simulink model "apilot1"  (Simulink 2.09)
settings: Solver=ode15s  StartTime=0.0  StopTime=100  MaxStep=2  RelTol=1e-06  AbsTol=1e-04
values from neighbouring files (symbols this model uses):
  ymod1A = [1 1 1 0 0]'    [apmode.m]
  ymod1S = [1 1 1 0 0]'    [apmode.m]
  yrefA = [0 Dpsir]'    [apmode.m]
  yrefS = [0 0 DHdotr]'    [apmode.m]
undefined symbols (not defined in the file or in its folder): Aail, Aelv, AM, Arud, Bail, Belv, Brud, Cail, Celv, Crud, Dail, Delv, Drud, GM1, sfunyst, uaero0, uprop0, xdot0, xfix, xinco
(part 1 of 2)
settings Model: SaveTime=off  SaveOutput=off  ConsistencyChecking=off  RTWTemplateMakefile=grt_vc.tmf

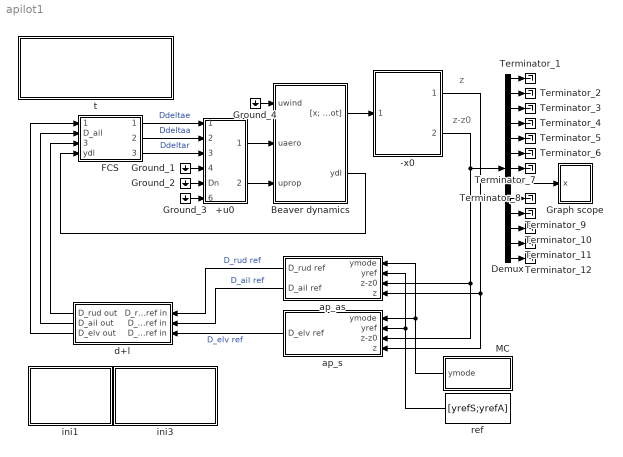
== system apilot1 ==
  note: z-z0
  note: z
  +u0 : Subsystem
      mask Display: disp('Add\ninitial\ninputs')
  -x0 : Subsystem
      mask Display: disp('Subtract\ninitial con-\nditions\n\nNo sensors!')
  Beaver dynamics : Subsystem
  Demux : Demux  Outputs=13
  FCS : Subsystem
      mask Display: disp('Actuator &\ncable dy-\nnamics')
  Graph scope : Subsystem  mask(Storage scope.){npts=100, color='g-'}
      mask prompts: npts "Initial Time Range:"; color "Initial y-min:"
      mask help:
      | Storage scope using MATLAB graph window.
      | Enter plotting ranges and line type.
      mask init:
      | close all; ax = [0, @1, @2, @3];
      mask Help: Uses MATLAB's graph window.\nUse only one block per system.\nLine type must be in quotes.\nSee the M-file sfunyst.m.
      mask Display: plot(0,0,100,100,[83,76,63,52,42,38,28,16,11,84,11,11,11,90,90,11],[75,58,47,54,72,80,84,74,65,65,65,90,40,40,90,90])
  Ground_{1..4} (4 alike) : Ground
  MC : Subsystem  Orientation=left
      mask Display: disp('Mode\nController')
  Terminator_{1..12} (12 alike) : Terminator
  ap_as : Subsystem  Orientation=left
      mask Display: disp('Asymmetrical\nautopilot modes')
  ap_s : Subsystem  Orientation=left
      mask Display: disp('Symmetrical\nautopilot modes')
  d+l : Subsystem  Orientation=left
      mask Display: disp('computational\ndelay & limiters')
  ini1 : Subsystem
      settings: OpenFcn=apinit
      mask Type: apinit
      mask Display: disp('1. Initialize\nsubsystems\n\nAPINIT')
  ini3 : Subsystem
      settings: OpenFcn=apmode
      mask Type: apmode
      mask Display: disp('2. Select mode &\nreference signals\n\nAPMODE')
  ref : Constant  Orientation=left  Value=[yrefS;yrefA]
      mask Display: disp('Reference\nsignals')
  t : Subsystem
      settings: OpenFcn=fdchelp apilot
      mask Display: disp('Apilot1 (no radio-navigation,\nwind, turbulence, and\nsensor models)\nMarc Rauw, June 2000')
  wires:
  +u0/2(uprop) -> Beaver dynamics/3(uprop)
  +u0/1(uaero) -> Beaver dynamics/2(uaero)
  Beaver dynamics/1("[x; Hdot]") -> -x0/1("[x; Hdot]")
  FCS/3(Ddeltar) -> +u0/3(Ddeltar)  "Ddeltar"
  FCS/2(Ddeltaa) -> +u0/2(Ddeltaa)  "Ddeltaa"
  FCS/1(Ddeltae) -> +u0/1(Ddeltae)  "Ddeltae"
  d+l/1(D_rud out) -> FCS/3(D_rud)
  d+l/2(D_ail out) -> FCS/2(D_ail)
  d+l/3(D_elv out) -> FCS/1(D_elv)
  ap_s/1(D_elv ref) -> d+l/3(D_elv ref in)  "D_elv ref"
  -x0/1("z == [x; Hdot] ") -> ap_s/4(z), ap_as/4(z)
  ref/1 -> ap_as/2(yref), ap_s/2(yref)
  -x0/2(z-z0 == [x-x0; Hdot-Hdot0]) -> ap_s/3(z-z0), ap_as/3(z-z0), Demux/1
  ap_as/1(D_rud ref) -> d+l/1(D_rud ref in)  "D_rud ref"
  ap_as/2(D_ail ref) -> d+l/2(D_ail ref in)  "D_ail ref"
  Beaver dynamics/2(ydl) -> FCS/4(ydl)
  MC/1(ymode) -> ap_as/1(ymode), ap_s/1(ymode)
  Demux/8 -> Graph scope/1(x)
  Ground_1/1 -> +u0/4(Ddeltaf)
  Ground_2/1 -> +u0/5(Dn)
  Ground_3/1 -> +u0/6(Dpz)
  Demux/1 -> Terminator_1/1
  Demux/2 -> Terminator_2/1
  Demux/3 -> Terminator_3/1
  Demux/4 -> Terminator_4/1
  Demux/5 -> Terminator_5/1
  Demux/6 -> Terminator_6/1
  Demux/7 -> Terminator_7/1
  Demux/9 -> Terminator_8/1
  Demux/10 -> Terminator_9/1
  Demux/11 -> Terminator_10/1
  Demux/12 -> Terminator_11/1
  Demux/13 -> Terminator_12/1
  Ground_4/1 -> Beaver dynamics/1(uwind)

== system apilot1/+u0 ==
  note: Add initial inputs
  note: ENGINE INPUTS:
  note: AERODYNAMIC INPUTS:
  Ddeltae : Inport  Port=1  PortWidth=-1  SampleTime=-1
  Ddeltaa : Inport  Port=2  PortWidth=-1  SampleTime=-1
  Ddeltar : Inport  Port=3  PortWidth=-1  SampleTime=-1
  Ddeltaf : Inport  Port=4  PortWidth=-1  SampleTime=-1
  Dn : Inport  Port=5  PortWidth=-1  SampleTime=-1
  Dpz : Inport  Port=6  PortWidth=-1  SampleTime=-1
  Initial inputs for aeromod : Constant  Value=uaero0
  Initial inputs for engmod : Constant  Value=uprop0
  Mux1 : Mux  Inputs=4
  Mux2 : Mux  Inputs=2
  Sum : Sum  Inputs=++
  Sum1 : Sum  Inputs=++
  uaero : Outport  Port=1  InitialOutput=0
  uprop : Outport  Port=2  InitialOutput=0
  wires:
  Dpz/1 -> Mux2/2
  Dn/1 -> Mux2/1
  Initial inputs for engmod/1 -> Sum/2
  Mux2/1 -> Sum/1
  Sum/1 -> uprop/1
  Ddeltaa/1 -> Mux1/2
  Ddeltae/1 -> Mux1/1
  Ddeltar/1 -> Mux1/3
  Ddeltaf/1 -> Mux1/4
  Initial inputs for aeromod/1 -> Sum1/1
  Sum1/1 -> uaero/1
  Mux1/1 -> Sum1/2

== system apilot1/-x0 ==
  note: Subtract initial conditions
  "[x; Hdot]" : Inport  Port=1  PortWidth=-1  SampleTime=-1
  Initial condition : Constant  Value=[xinco; xdot0(12)]
  Sum : Sum  Inputs=+-
  "z == [x; Hdot] " : Outport  Port=1  InitialOutput=0
  z-z0 == [x-x0; Hdot-Hdot0] : Outport  Port=2  InitialOutput=0
  wires:
  "[x; Hdot]"/1 -> "z == [x; Hdot] "/1, Sum/1
  Initial condition/1 -> Sum/2
  Sum/1 -> z-z0 == [x-x0; Hdot-Hdot0]/1

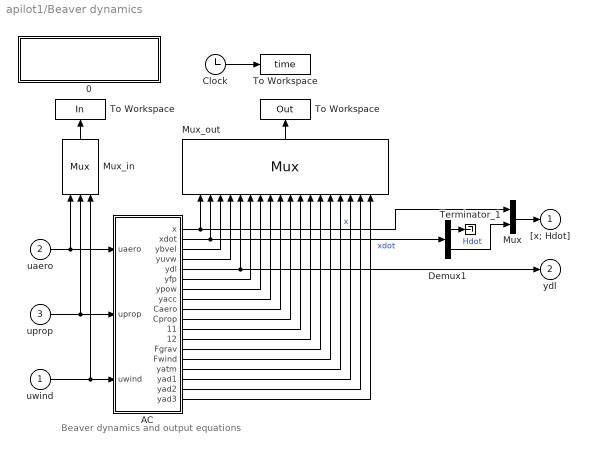
== system apilot1/Beaver dynamics ==
  note: Beaver dynamics
      | and output equations
  uwind : Inport  Port=1  PortWidth=6  SampleTime=-1
  uaero : Inport  Port=2  PortWidth=4  SampleTime=-1
  uprop : Inport  Port=3  PortWidth=2  SampleTime=-1
  0 : Subsystem
      settings: OpenFcn=fdchelp level1
      mask Display: disp('Subsystem equivalent of\nthe S-function BEAVER\nM.O. Rauw, October 1997')
  AC : Subsystem
  Clock : Clock
  Demux1 : Demux  Outputs=[11 1]
  Mux : Mux  Inputs=[12 1]
  Mux_in : Mux  Orientation=up  Inputs=[4 2 6]
      settings: OpenFcn=fdchelp inputs
      mask Display: disp('Mux\nclick\n2x for\ninfo!')
  Mux_out : Mux  Orientation=up  Inputs=[12 12 3 3 3 4 2 6 6 6 6 6 3 3 5 3 3 3]
      settings: OpenFcn=fdchelp outputs
      mask Display: disp('Mux\n\nDouble-click for info!')
  Terminator_1 : Terminator
  To Workspace : ToWorkspace  VariableName=Out  SampleTime=0
      settings: Orientation=up  Buffer=5000
  "To Workspace " : ToWorkspace  VariableName=In  SampleTime=0
      settings: Orientation=up  Buffer=5000
  "To Workspace  " : ToWorkspace  VariableName=time  SampleTime=0
      settings: Buffer=5000
  "[x; Hdot]" : Outport  Port=1  InitialOutput=0
  ydl : Outport  Port=2  InitialOutput=0
  wires:
  AC/7(ypow) -> Mux_out/7
  Mux_in/1 -> "To Workspace "/1
  Mux_out/1 -> To Workspace/1
  Clock/1 -> "To Workspace  "/1
  AC/2(xdot) -> Mux_out/2, Demux1/1  "xdot"
  AC/15(yatm) -> Mux_out/15
  AC/14(Fwind) -> Mux_out/14
  AC/13(Fgrav) -> Mux_out/13
  AC/12(FMprop) -> Mux_out/12
  AC/11(FMaero) -> Mux_out/11
  AC/10(Cprop) -> Mux_out/10
  AC/9(Caero) -> Mux_out/9
  AC/8(yacc) -> Mux_out/8
  AC/6(yfp) -> Mux_out/6
  AC/5(ydl) -> ydl/1, Mux_out/5
  AC/16(yad1) -> Mux_out/16
  AC/3(ybvel) -> Mux_out/3
  AC/1(x) -> Mux/1, Mux_out/1  "x"
  AC/4(yuvw) -> Mux_out/4
  AC/17(yad2) -> Mux_out/17
  AC/18(yad3) -> Mux_out/18
  uwind/1 -> AC/3(" uwind"), Mux_in/3
  uprop/1 -> AC/2(uprop), Mux_in/2
  uaero/1 -> AC/1(uaero), Mux_in/1
  Demux1/1 -> Terminator_1/1
  Demux1/2 -> Mux/2  "Hdot"
  Mux/1 -> "[x; Hdot]"/1

== system apilot1/FCS ==
  note: Actuators
      | + cables:
  D_elv : Inport  Port=1  PortWidth=-1  SampleTime=-1
  D_ail : Inport  Port=2  PortWidth=-1  SampleTime=-1
  D_rud : Inport  Port=3  PortWidth=-1  SampleTime=-1
  ydl : Inport  Port=4  PortWidth=-1  SampleTime=-1
  Demux1 : Demux  Outputs=3
  Mux1 : Mux  Inputs=2
  Mux2 : Mux  Inputs=2
  Mux3 : Mux  Inputs=2
  ailerons : StateSpace  A=Aail  B=Bail  C=Cail*2  D=Dail  X0=0
  elevator : StateSpace  A=Aelv  B=Belv  C=Celv  D=Delv  X0=0
  rudder : StateSpace  A=Arud  B=Brud  C=Crud  D=Drud  X0=0
  t : Subsystem
      settings: OpenFcn=fdchelp actuatr
      mask Display: disp('Actuator & cable dynamics\nMarc Rauw, October 1997')
  Ddeltae : Outport  Port=1  InitialOutput=0
  Ddeltaa : Outport  Port=2  InitialOutput=0
  Ddeltar : Outport  Port=3  InitialOutput=0
  wires:
  Demux1/2 -> Mux1/2
  Demux1/1 -> Mux2/2
  Demux1/3 -> Mux3/2
  Mux1/1 -> elevator/1
  Mux2/1 -> ailerons/1
  Mux3/1 -> rudder/1
  elevator/1 -> Ddeltae/1
  ailerons/1 -> Ddeltaa/1
  ydl/1 -> Demux1/1
  rudder/1 -> Ddeltar/1
  D_elv/1 -> Mux1/1
  D_ail/1 -> Mux2/1
  D_rud/1 -> Mux3/1

== system apilot1/Graph scope ==
  x : Inport  Port=1  PortWidth=-1  SampleTime=-1
  "S-function M-file which plots lines " : S-Function  LoadFcn=sfunyst([],[],[],'LoadBlock')  FunctionName=sfunyst  Parameters=ax, color, npts
      settings: CopyFcn=sfunyst([],[],[],'CopyBlock')  DeleteFcn=sfunyst([],[],[],'DeleteBlock')
  wires:
  x/1 -> "S-function M-file which plots lines "/1

== system apilot1/MC ==
  Mux1 : Mux  Inputs=[5 5]
  asymm. mode-switches : Constant  Value=ymod1A
  symm. mode-switches : Constant  Value=ymod1S
  t : Subsystem
      settings: OpenFcn=fdchelp modectrl
      mask Display: disp('Mode Controller (Mode Select)\nNo on-line mode-switching!\nMarc Rauw, June 2000')
  ymode : Outport  Port=1  InitialOutput=0
  wires:
  symm. mode-switches/1 -> Mux1/1
  Mux1/1 -> ymode/1
  asymm. mode-switches/1 -> Mux1/2

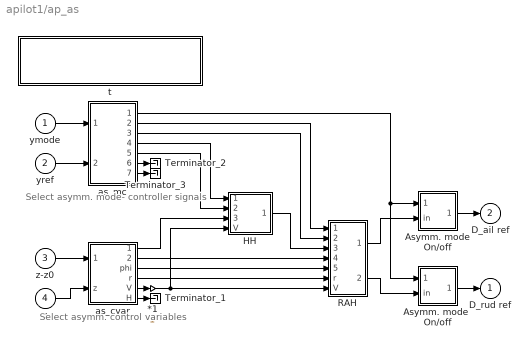
== system apilot1/ap_as ==
  note: Select asymm. mode-
      | controller signals
  note: Select asymm.
      | control variables
  ymode : Inport  Port=1  PortWidth=-1  SampleTime=-1
  yref : Inport  Port=2  PortWidth=-1  SampleTime=-1
  z-z0 : Inport  Port=3  PortWidth=-1  SampleTime=-1
  z : Inport  Port=4  PortWidth=-1  SampleTime=-1
  *1 : Gain  Gain=1
  Asymm. mode On/off : Subsystem
      mask Type: On/off switch
      mask Description:
      | If input(1) = 1
      |      output = input(2)
      |  else if input(1) = 0
      |      output = 0
      mask Help: On/off switch.
      mask Display: plot(0,0,100,100,[31,31,32,34,34,32,31,31,0],[50,48,47,48,51,53,51,50,50],[100,75,51],[50,50,97]);disp('?')
  Asymm. mode  On/off : Subsystem
      mask Type: On/off switch
      mask Description:
      | If input(1) = 1
      |      output = input(2)
      |  else if input(1) = 0
      |      output = 0
      mask Help: On/off switch.
      mask Display: plot(0,0,100,100,[31,31,32,34,34,32,31,31,0],[50,48,47,48,51,53,51,50,50],[100,75,51],[50,50,97]);disp('?')
  HH : Subsystem
  RAH : Subsystem
  Terminator_1 : Terminator
  Terminator_2 : Terminator
  Terminator_3 : Terminator
  as_cvar : Subsystem
  as_mc : Subsystem
  t : Subsystem
      settings: OpenFcn=fdchelp ap_asymm
      mask Display: disp('Asymm. autopilot modes\n(without NAV and LOC modes)\nMarc Rauw, October 1997')
  D_rud ref : Outport  Port=1  InitialOutput=0
  D_ail ref : Outport  Port=2  InitialOutput=0
  wires:
  *1/1 -> RAH/7(V), HH/4(V)
  RAH/2(D_rud ref) -> Asymm. mode  On/off/2(in)
  ymode/1 -> as_mc/1(ymode)
  yref/1 -> as_mc/2(yref)
  Asymm. mode On/off/1(out) -> D_ail ref/1
  Asymm. mode  On/off/1(out) -> D_rud ref/1
  z-z0/1 -> as_cvar/1(z-z0)
  as_cvar/5(V) -> *1/1
  as_cvar/2(phi-phi0) -> RAH/4(phi-phi0)
  as_cvar/3(phi) -> RAH/5(phi)
  as_cvar/4(r) -> RAH/6(r)
  z/1 -> as_cvar/2(z)
  HH/1(Dphir (HH)) -> RAH/3(Dphir (out. loop))
  as_cvar/1(psi-psi0) -> HH/3(psi-psi0)
  RAH/1(D_ail ref) -> Asymm. mode On/off/2(in)
  as_mc/1(asymm. mode?) -> Asymm. mode  On/off/1(crit), Asymm. mode On/off/1(crit)
  as_mc/2(asymm. out. loop?) -> RAH/1(Asymm out. loop?)
  as_mc/3(Dphir (RAH)) -> RAH/2(Dphir (RAH))
  as_mc/4(HH?) -> HH/1(HH?)
  as_mc/5(Dpsir (HH)) -> HH/2(Dpsir (HH))
  as_cvar/6(H) -> Terminator_1/1
  as_mc/6(NAV?) -> Terminator_2/1
  as_mc/7(LOC coupled?) -> Terminator_3/1

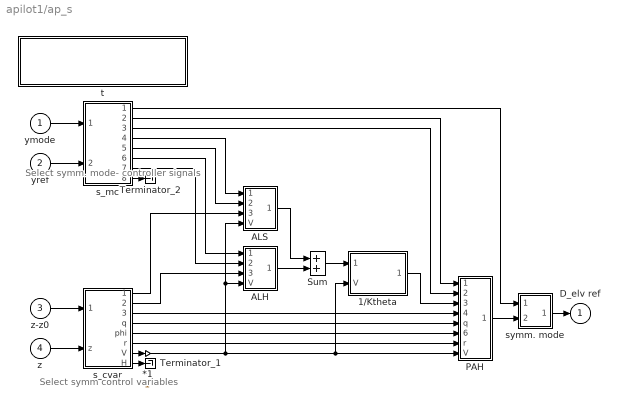
== system apilot1/ap_s ==
  note: Select symm
      | control variables
  note: Select symm. mode-
      | controller signals
  ymode : Inport  Port=1  PortWidth=-1  SampleTime=-1
  yref : Inport  Port=2  PortWidth=-1  SampleTime=-1
  z-z0 : Inport  Port=3  PortWidth=-1  SampleTime=-1
  z : Inport  Port=4  PortWidth=-1  SampleTime=-1
  *1 : Gain  Gain=1
  1/Ktheta : Subsystem
      mask Display: plot(0,0,100,100,[0,100,0],[0,50,100]);disp('K(u1)      ')
  ALH : Subsystem
  ALS : Subsystem
  PAH : Subsystem
  Sum : Sum  Inputs=++
  Terminator_1 : Terminator
  Terminator_2 : Terminator
  s_cvar : Subsystem
  s_mc : Subsystem
  symm. mode : Subsystem
      mask Type: On/off switch
      mask Description:
      | If input(1) = 1
      |      output = input(2)
      |  else if input(1) = 0
      |      output = 0
      mask Help: On/off switch. \nIf input(1) = 1, the output equals input(1). \nIf input(1) = 0, the output is zero.
      mask Display: plot(0,0,100,100,[31,31,32,34,34,32,31,31,0],[50,48,47,48,51,53,51,50,50],[100,75,51],[50,50,97]);disp('?')
  t : Subsystem
      settings: OpenFcn=fdchelp ap_symm
      mask Display: disp('Symm. autopilot modes\n(without glideslope mode)\nMarc Rauw, October 1997')
  D_elv ref : Outport  Port=1  InitialOutput=0
  wires:
  Sum/1 -> 1/Ktheta/1(input u)
  symm. mode/1(out) -> D_elv ref/1
  PAH/1(D_elv ref) -> symm. mode/2(in)
  ALH/1(Dthetar (ALH)) -> Sum/2
  s_cvar/2(H-H0) -> ALH/3(H-H0)
  s_cvar/3(theta-theta0) -> PAH/4(theta-theta0)
  s_cvar/4(q) -> PAH/5(q)
  s_cvar/5(phi) -> PAH/6(phi)
  s_cvar/6(r) -> PAH/7(r)
  s_cvar/7(V) -> *1/1
  z-z0/1 -> s_cvar/1(z-z0)
  z/1 -> s_cvar/2(z)
  s_mc/4(ALS?) -> ALS/1(ALS?)
  s_mc/5(DHdot r (ALS)) -> ALS/2(DHdot r (ALS))
  s_mc/6(ALH?) -> ALH/1(ALH?)
  s_mc/7(DHr (ALH)) -> ALH/2(DHr (ALH))
  ymode/1 -> s_mc/1(ymode)
  yref/1 -> s_mc/2(yref)
  s_mc/3(Dthetar (PAH)) -> PAH/2(Dthetar (PAH/GA))
  s_mc/2(symm. outer loop?) -> PAH/1(Symm out. loop?)
  s_mc/1(symm mode?) -> symm. mode/1(crit)
  s_cvar/1(Hdot-Hdot0) -> ALS/3(Hdot-Hdot0)
  *1/1 -> PAH/8(V), 1/Ktheta/2(V), ALS/4(V), ALH/4(V)
  ALS/1(Dthetar (ALS)) -> Sum/1
  1/Ktheta/1(y = K*u) -> PAH/3(Dthetar (out. loop))
  s_cvar/8(H) -> Terminator_1/1
  s_mc/8(GS coupled?) -> Terminator_2/1

== system apilot1/d+l ==
  D_rud ref in : Inport  Port=1  PortWidth=-1  SampleTime=-1
  D_ail ref in : Inport  Port=2  PortWidth=-1  SampleTime=-1
  D_elv ref in : Inport  Port=3  PortWidth=-1  SampleTime=-1
  " +/- 10 V " : Saturate  UpperLimit=10 * (pi/180)  LowerLimit=-10 * (pi/180)
  " delay" : TransportDelay  DelayTime=0.03  InitialInput=0  BufferSize=1024
  +/- 10 V : Saturate  UpperLimit=10 * (pi/180)  LowerLimit=-10 * (pi/180)
  "+/- 10 V " : Saturate  UpperLimit=10 * (pi/180)  LowerLimit=-10 * (pi/180)
  delay : TransportDelay  DelayTime=0.03  InitialInput=0  BufferSize=1024
  "delay " : TransportDelay  DelayTime=0.03  InitialInput=0  BufferSize=1024
  t : Subsystem
      settings: OpenFcn=fdchelp delaylim
      mask Display: disp('Computational delay and\ninput limiters (+- 10 Volt)\nMarc Rauw, October 1997')
  D_rud out : Outport  Port=1  InitialOutput=0
  D_ail out : Outport  Port=2  InitialOutput=0
  D_elv out : Outport  Port=3  InitialOutput=0
  wires:
  D_rud ref in/1 -> delay/1
  delay/1 -> +/- 10 V/1
  D_elv ref in/1 -> " delay"/1
  " +/- 10 V "/1 -> D_elv out/1
  D_ail ref in/1 -> "delay "/1
  "+/- 10 V "/1 -> D_ail out/1
  +/- 10 V/1 -> D_rud out/1
  " delay"/1 -> " +/- 10 V "/1
  "delay "/1 -> "+/- 10 V "/1

== system apilot1/ini1 ==

== system apilot1/ini3 ==

== system apilot1/t ==

== system apilot1/Beaver dynamics/0 ==

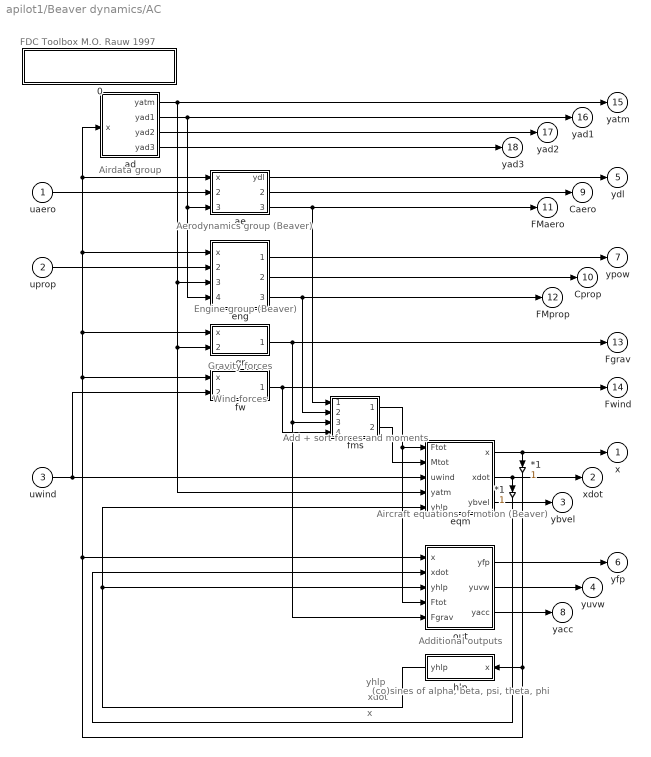
== system apilot1/Beaver dynamics/AC ==
  note: FDC Toolbox
      |  M.O. Rauw 1997
  note: xdot
  note: x
  note: yhlp
  note: Additional outputs
  note: Aircraft equations
      | of motion (Beaver)
  note: Wind forces
  note: Gravity forces
  note: Engine group (Beaver)
  note: Aerodynamics
      | group (Beaver)
  note: (co)sines of
      | alpha, beta,
      | psi, theta, phi
  note: Add + sort
      | forces and
      | moments
  note: Airdata group
  uaero : Inport  Port=1  PortWidth=-1  SampleTime=-1
  uprop : Inport  Port=2  PortWidth=-1  SampleTime=-1
  " uwind" : Inport  Port=3  PortWidth=-1  SampleTime=-1
  " *1" : Gain  Orientation=down  Gain=1
  *1 : Gain  Orientation=down  Gain=1
  0 : Subsystem
      settings: OpenFcn=fdchelp level2
      mask Display: disp('BEAVER, level 2 (main level)\nM.O. Rauw')
  ad : Subsystem
  ae : Subsystem
  eng : Subsystem
  eqm : Subsystem
  fms : Subsystem
      mask Type: FMsort
      mask Description: Forces and Moments sorting block
      mask Help: eval('fdchelp fmsort')
      mask Display: disp('FMsort')
  fw : Subsystem  mask(fwind){m=GM1(10)}
      mask prompts: m "Mass of the aircraft [kg]:"
      mask help: Forces due to non-steady atmosphere.
      mask Help: eval('fdchelp fwind')
      mask Display: disp('Fwind')
  gr : Subsystem  mask(Gravity){m=GM1(10)}
      mask prompts: m "Mass of the aircraft [kg]:"
      mask help: Gravity forces.
      mask Help: eval('fdchelp gravity')
      mask Display: disp('Gravity')
  hlp : Subsystem  Orientation=left
      mask Type: Hlpfcn
      mask Description: Help sines and cosines
      mask Help: eval('fdchelp hlpfcn')
      mask Display: disp('hlpfcn')
  out : Subsystem
  x : Outport  Port=1  InitialOutput=0
  xdot : Outport  Port=2  InitialOutput=0
  ybvel : Outport  Port=3  InitialOutput=0
  yuvw : Outport  Port=4  InitialOutput=0
  ydl : Outport  Port=5  InitialOutput=0
  yfp : Outport  Port=6  InitialOutput=0
  ypow : Outport  Port=7  InitialOutput=0
  yacc : Outport  Port=8  InitialOutput=0
  Caero : Outport  Port=9  InitialOutput=0
  Cprop : Outport  Port=10  InitialOutput=0
  FMaero : Outport  Port=11  InitialOutput=0
  FMprop : Outport  Port=12  InitialOutput=0
  Fgrav : Outport  Port=13  InitialOutput=0
  Fwind : Outport  Port=14  InitialOutput=0
  yatm : Outport  Port=15  InitialOutput=0
  yad1 : Outport  Port=16  InitialOutput=0
  yad2 : Outport  Port=17  InitialOutput=0
  yad3 : Outport  Port=18  InitialOutput=0
  wires:
  out/2(yuvw) -> yuvw/1
  uprop/1 -> eng/2(uprop)
  uaero/1 -> ae/2(uaero)
  ad/4(yad3) -> yad3/1
  ae/1(ydl) -> ydl/1
  ae/2(Caero) -> Caero/1
  eng/1(ypow) -> ypow/1
  eng/2(Cprop) -> Cprop/1
  eqm/3(ybvel) -> ybvel/1
  out/1(yfp) -> yfp/1
  ad/2(yad1) -> eng/4(yad1), ae/3(yad1), yad1/1
  ad/3(yad2) -> yad2/1
  ad/1(yatm) -> yatm/1, eng/3(yatm), eqm/4(yatm), gr/2(yatm)
  out/3(yacc) -> yacc/1
  fw/1(Fwind) -> Fwind/1, fms/4(Fwind)
  eng/3(FMprop) -> FMprop/1, fms/2(FMprop)
  ae/3(FMaero) -> FMaero/1, fms/1(FMaero)
  hlp/1(yhlp) -> eqm/5(yhlp), out/3(yhlp)
  " uwind"/1 -> eqm/3(uwind), fw/2(uwind)
  *1/1 -> out/2(xdot)
  gr/1(Fgrav) -> Fgrav/1, fms/3(Fgrav), out/5(Fgrav)
  " *1"/1 -> hlp/1(x), out/1(x), fw/1(x), gr/1(x), eng/1(x), ae/1(x), ad/1(x)
  eqm/2(xdot) -> xdot/1, *1/1
  eqm/1(x) -> x/1, " *1"/1
  fms/1(Ftot) -> out/4(Ftot), eqm/1(Ftot)
  fms/2(Mtot) -> eqm/2(Mtot)

== system apilot1/FCS/t ==

== system apilot1/MC/t ==

== system apilot1/ap_as/Asymm. mode On/off ==
  crit : Inport  Port=1  PortWidth=-1  SampleTime=-1
  in : Inport  Port=2  PortWidth=-1  SampleTime=-1
  Sum : Sum  Inputs=+-
  Switch : Switch  Threshold=0
  const. : Constant  Value=0.5
  const.1 : Constant  Value=0
  out : Outport  Port=1  InitialOutput=0
  wires:
  crit/1 -> Sum/1
  const.1/1 -> Switch/3
  Sum/1 -> Switch/2
  Switch/1 -> out/1
  in/1 -> Switch/1
  const./1 -> Sum/2

== system apilot1/ap_as/Asymm. mode  On/off ==
  crit : Inport  Port=1  PortWidth=-1  SampleTime=-1
  in : Inport  Port=2  PortWidth=-1  SampleTime=-1
  Sum : Sum  Inputs=+-
  Switch : Switch  Threshold=0
  const. : Constant  Value=0.5
  const.1 : Constant  Value=0
  out : Outport  Port=1  InitialOutput=0
  wires:
  const./1 -> Sum/2
  in/1 -> Switch/1
  Switch/1 -> out/1
  Sum/1 -> Switch/2
  const.1/1 -> Switch/3
  crit/1 -> Sum/1

== system apilot1/ap_as/HH ==
  note: Heading Hold / Heading Select mode
  HH? : Inport  Port=1  PortWidth=-1  SampleTime=-1
  Dpsir (HH) : Inport  Port=2  PortWidth=-1  SampleTime=-1
  psi-psi0 : Inport  Port=3  PortWidth=-1  SampleTime=-1
  V : Inport  Port=4  PortWidth=-1  SampleTime=-1
  Kpsi : Subsystem
      mask Display: plot(0,0,100,100,[0,100,0],[0,50,100]);disp('K(u1)      ')
  On/Off : Subsystem
      mask Type: On/off switch
      mask Description:
      | If input(1) = 1
      |      output = input(2)
      |  else if input(1) = 0
      |      output = 0
      mask Help: On/off switch.
      mask Display: plot(0,0,100,100,[31,31,32,34,34,32,31,31,0],[50,48,47,48,51,53,51,50,50],[100,75,51],[50,50,97]);disp('?')
  Sum : Sum  Inputs=+-
  Dphir (HH) : Outport  Port=1  InitialOutput=0
  wires:
  V/1 -> Kpsi/1(V)
  HH?/1 -> On/Off/1(crit)
  Dpsir (HH)/1 -> Sum/1
  psi-psi0/1 -> Sum/2
  Kpsi/1(y = K*u) -> On/Off/2(in)
  Sum/1 -> Kpsi/2(input u)
  On/Off/1(out) -> Dphir (HH)/1

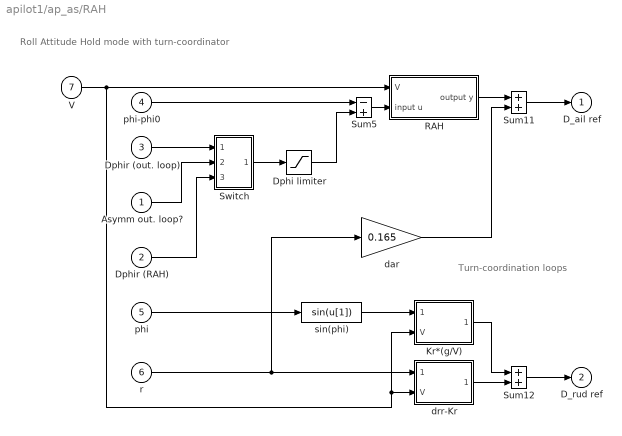
== system apilot1/ap_as/RAH ==
  note: Turn-coordination loops
  note: Roll Attitude Hold mode
      | with turn-coordinator
  Asymm out. loop? : Inport  Port=1  PortWidth=-1  SampleTime=-1
  Dphir (RAH) : Inport  Port=2  PortWidth=-1  SampleTime=-1
  Dphir (out. loop) : Inport  Port=3  PortWidth=-1  SampleTime=-1
  phi-phi0 : Inport  Port=4  PortWidth=-1  SampleTime=-1
  phi : Inport  Port=5  PortWidth=-1  SampleTime=-1
  r : Inport  Port=6  PortWidth=-1  SampleTime=-1
  V : Inport  Port=7  PortWidth=-1  SampleTime=-1
  Dphi limiter : Saturate  UpperLimit=30*pi/180  LowerLimit=-30*pi/180
  Kr*(g/V) : Subsystem
      mask Display: plot(0,0,100,100,[0,100,0],[0,50,100]);disp('K(u2)      ')
  RAH : Subsystem
      mask Display: disp('RAH (limited \n PI controller)')
  Sum11 : Sum  Inputs=++
  Sum12 : Sum  Inputs=++
  Sum5 : Sum  Inputs=-+
  Switch : Subsystem
      mask Display: plot(0,0,100,100,[100,70,40,0],[50,50,80,80],[40,0],[20,20],[29,29,0],[64,50,50],[29,29],[36,50],[40,40,41,40,39,40],[80,82,80,78,80,82],[40,40,41,40,39,40],[19,21,20,18,20,23])
  dar : Gain  Gain=0.165
  drr-Kr : Subsystem
      mask Display: plot(0,0,100,100,[0,100,0],[0,50,100]);disp('K(u2)      ')
  sin(phi) : Fcn  Expr=sin(u[1])
  D_ail ref : Outport  Port=1  InitialOutput=0
  D_rud ref : Outport  Port=2  InitialOutput=0
  wires:
  V/1 -> RAH/1(V), Kr*(g/V)/2(V), drr-Kr/2(V)
  phi/1 -> sin(phi)/1
  phi-phi0/1 -> Sum5/1
  Switch/1(Dphir) -> Dphi limiter/1
  RAH/1(output y) -> Sum11/1
  Sum11/1 -> D_ail ref/1
  Sum12/1 -> D_rud ref/1
  drr-Kr/1(y = K*u) -> Sum12/2
  sin(phi)/1 -> Kr*(g/V)/1(input u)
  Kr*(g/V)/1(y = K*u) -> Sum12/1
  dar/1 -> Sum11/2
  Sum5/1 -> RAH/2(input u)
  Dphi limiter/1 -> Sum5/2
  r/1 -> drr-Kr/1(input u), dar/1
  Dphir (out. loop)/1 -> Switch/1(Dphir (out. loop))
  Asymm out. loop?/1 -> Switch/2(Asymm.  out. loop?)
  Dphir (RAH)/1 -> Switch/3(Dphir (RAH))

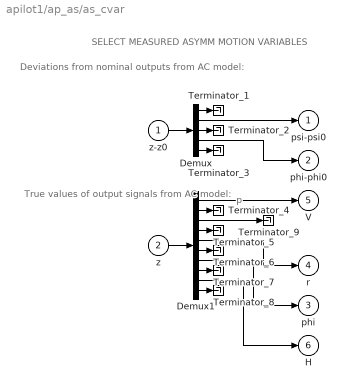
== system apilot1/ap_as/as_cvar ==
  note: p
  note: SELECT MEASURED ASYMM MOTION VARIABLES
  note: Deviations from nominal
      | outputs from AC model:
  note: True values of output
      | signals from AC model:
  z-z0 : Inport  Port=1  PortWidth=-1  SampleTime=-1
  z : Inport  Port=2  PortWidth=-1  SampleTime=-1
  Demux : Demux  Outputs=[6 1 1 1 4]
  Demux1 : Demux  Outputs=[1 2 1 1 1 2 1 2 1 1]
  Terminator_{1..9} (9 alike) : Terminator
  psi-psi0 : Outport  Port=1  InitialOutput=0
  phi-phi0 : Outport  Port=2  InitialOutput=0
  phi : Outport  Port=3  InitialOutput=0
  r : Outport  Port=4  InitialOutput=0
  V : Outport  Port=5  InitialOutput=0
  H : Outport  Port=6  InitialOutput=0
  wires:
  z-z0/1 -> Demux/1
  Demux/2 -> psi-psi0/1
  Demux/4 -> phi-phi0/1
  Demux/1 -> Terminator_1/1
  Demux/3 -> Terminator_2/1
  Demux/5 -> Terminator_3/1
  Demux1/9 -> H/1
  z/1 -> Demux1/1
  Demux1/3 -> Terminator_9/1
  Demux1/5 -> r/1
  Demux1/7 -> phi/1
  Demux1/2 -> Terminator_4/1
  Demux1/4 -> Terminator_5/1
  Demux1/6 -> Terminator_6/1
  Demux1/8 -> Terminator_7/1
  Demux1/10 -> Terminator_8/1
  Demux1/1 -> V/1

== system apilot1/ap_as/as_mc ==
  note: SELECT ASYMM MODE (on/off flags denoted by '?')
  note: SELECT ASYMM REFERENCE SIGNALS
  ymode : Inport  Port=1  PortWidth=-1  SampleTime=-1
  yref : Inport  Port=2  PortWidth=-1  SampleTime=-1
  Demux : Demux  Outputs=[5 1 1 1 1 1]
  Demux1 : Demux  Outputs=[3 1 1]
  Terminator_1 : Terminator
  Terminator_2 : Terminator
  asymm. mode? : Outport  Port=1  InitialOutput=0
  asymm. out. loop? : Outport  Port=2  InitialOutput=0
  Dphir (RAH) : Outport  Port=3  InitialOutput=0
  HH? : Outport  Port=4  InitialOutput=0
  Dpsir (HH) : Outport  Port=5  InitialOutput=0
  NAV? : Outport  Port=6  InitialOutput=0
  LOC coupled? : Outport  Port=7  InitialOutput=0
  wires:
  yref/1 -> Demux1/1
  Demux1/2 -> Dphir (RAH)/1
  Demux1/3 -> Dpsir (HH)/1
  ymode/1 -> Demux/1
  Demux/2 -> asymm. mode?/1
  Demux/3 -> asymm. out. loop?/1
  Demux/4 -> HH?/1
  Demux/5 -> NAV?/1
  Demux/6 -> LOC coupled?/1
  Demux/1 -> Terminator_1/1
  Demux1/1 -> Terminator_2/1

== system apilot1/ap_as/t ==

== system apilot1/ap_s/1/Ktheta ==
  input u : Inport  Port=1  PortWidth=-1  SampleTime=-1
  V : Inport  Port=2  PortWidth=-1  SampleTime=-1
  1/Ktheta : Fcn  Expr=1/(-1.375*10^(-3)*u[1]^2 + 0.1575*u[1] - 4.8031)
  Product : Product  Inputs=2
  y = K*u : Outport  Port=1  InitialOutput=0
  wires:
  V/1 -> 1/Ktheta/1
  Product/1 -> y = K*u/1
  input u/1 -> Product/2
  1/Ktheta/1 -> Product/1

== system apilot1/ap_s/ALH ==
  note: Altitude Hold mode
  ALH? : Inport  Port=1  PortWidth=-1  SampleTime=-1
  DHr (ALH) : Inport  Port=2  PortWidth=-1  SampleTime=-1
  H-H0 : Inport  Port=3  PortWidth=-1  SampleTime=-1
  V : Inport  Port=4  PortWidth=-1  SampleTime=-1
  KH : Subsystem
      mask Display: plot(0,0,100,100,[0,100,0],[0,50,100]);disp('K(u1)      ')
  On/Off : Subsystem
      mask Type: On/off switch
      mask Description:
      | If input(1) = 1
      |      output = input(2)
      |  else if input(1) = 0
      |      output = 0
      mask Help: On/off switch.
      mask Display: plot(0,0,100,100,[31,31,32,34,34,32,31,31,0],[50,48,47,48,51,53,51,50,50],[100,75,51],[50,50,97]);disp('?')
  Sum : Sum  Inputs=+-
  Dthetar (ALH) : Outport  Port=1  InitialOutput=0
  wires:
  V/1 -> KH/1(V)
  Sum/1 -> KH/2(input u)
  KH/1(y = K*u) -> On/Off/2(in)
  ALH?/1 -> On/Off/1(crit)
  DHr (ALH)/1 -> Sum/1
  On/Off/1(out) -> Dthetar (ALH)/1
  H-H0/1 -> Sum/2

== system apilot1/ap_s/ALS ==
  note: Altitude Select Mode
  ALS? : Inport  Port=1  PortWidth=-1  SampleTime=-1
  DHdot r (ALS) : Inport  Port=2  PortWidth=-1  SampleTime=-1
  Hdot-Hdot0 : Inport  Port=3  PortWidth=-1  SampleTime=-1
  V : Inport  Port=4  PortWidth=-1  SampleTime=-1
  KHdot : Subsystem
      mask Display: plot(0,0,100,100,[0,100,0],[0,50,100]);disp('K(u1)      ')
  On/Off : Subsystem
      mask Type: On/off switch
      mask Description:
      | If input(1) = 1
      |      output = input(2)
      |  else if input(1) = 0
      |      output = 0
      mask Help: On/off switch.
      mask Display: plot(0,0,100,100,[31,31,32,34,34,32,31,31,0],[50,48,47,48,51,53,51,50,50],[100,75,51],[50,50,97]);disp('?')
  Sum : Sum  Inputs=+-
  filter : TransferFcn  Numerator=[1]  Denominator=[1 0.15]
  Dthetar (ALS) : Outport  Port=1  InitialOutput=0
  wires:
  V/1 -> KHdot/1(V)
  Hdot-Hdot0/1 -> Sum/2
  KHdot/1(y = K*u) -> On/Off/2(in)
  ALS?/1 -> On/Off/1(crit)
  DHdot r (ALS)/1 -> Sum/1
  On/Off/1(out) -> Dthetar (ALS)/1
  Sum/1 -> filter/1
  filter/1 -> KHdot/2(input u)

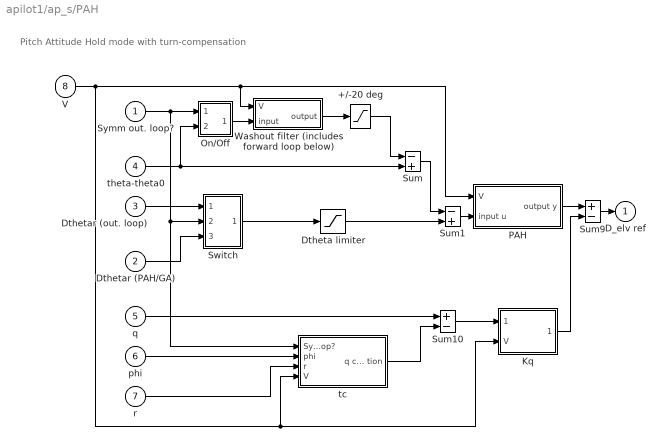
== system apilot1/ap_s/PAH ==
  note: Pitch Attitude Hold mode
      | with turn-compensation
  Symm out. loop? : Inport  Port=1  PortWidth=-1  SampleTime=-1
  Dthetar (PAH/GA) : Inport  Port=2  PortWidth=-1  SampleTime=-1
  Dthetar (out. loop) : Inport  Port=3  PortWidth=-1  SampleTime=-1
  theta-theta0 : Inport  Port=4  PortWidth=-1  SampleTime=-1
  q : Inport  Port=5  PortWidth=-1  SampleTime=-1
  phi : Inport  Port=6  PortWidth=-1  SampleTime=-1
  r : Inport  Port=7  PortWidth=-1  SampleTime=-1
  V : Inport  Port=8  PortWidth=-1  SampleTime=-1
  +/-20 deg : Saturate  UpperLimit=20*(pi/180)  LowerLimit=-20*(pi/180)
  Dtheta limiter : Saturate  UpperLimit=18*(pi/180)  LowerLimit=-8*(pi/180)
  Kq : Subsystem
      mask Display: plot(0,0,100,100,[0,100,0],[0,50,100]);disp('K(u2)      ')
  On/Off : Subsystem
      mask Type: On/off switch
      mask Description:
      | If input(1) = 1
      |      output = input(2)
      |  else if input(1) = 0
      |      output = 0
      mask Help: On/off switch. \nIf input(1) = 1, the output equals input(2). \nIf input(1) = 0, the output is zero.
      mask Display: plot(0,0,100,100,[31,31,32,34,34,32,31,31,0],[50,48,47,48,51,53,51,50,50],[100,75,51],[50,50,97]);disp('?')
  PAH : Subsystem
      mask Display: disp('PAH (limited \n PI controller)')
  Sum : Sum  Inputs=-+
  Sum1 : Sum  Inputs=-+
  Sum10 : Sum  Inputs=+-
  Sum9 : Sum  Inputs=+-
  Switch : Subsystem
      mask Display: plot(0,0,100,100,[100,70,40,0],[50,50,80,80],[40,0],[20,20],[29,29,0],[64,50,50],[29,29],[36,50],[40,40,41,40,39,40],[80,82,80,78,80,82],[40,40,41,40,39,40],[19,21,20,18,20,23])
  Washout filter (includes forward loop below) : Subsystem
      mask Display: disp('Kd/(s+Kd)')
  tc : Subsystem
      mask Display: disp('Turn\nCompensator')
  D_elv ref : Outport  Port=1  InitialOutput=0
  wires:
  Symm out. loop?/1 -> On/Off/1(crit.), tc/1(Symm. outer loop?), Switch/2(Symm.  out. loop?)
  Dthetar (out. loop)/1 -> Switch/1(Dthetar (out. loop))
  Switch/1(Dthetar) -> Dtheta limiter/1
  r/1 -> tc/3(r)
  phi/1 -> tc/2(phi)
  Washout filter (includes forward loop below)/1(output) -> +/-20 deg/1
  On/Off/1(out) -> Washout filter (includes forward loop below)/2(input)
  Sum9/1 -> D_elv ref/1
  Sum1/1 -> PAH/2(input u)
  Dtheta limiter/1 -> Sum1/2
  PAH/1(output y) -> Sum9/1
  Sum10/1 -> Kq/1(input u)
  q/1 -> Sum10/1
  Kq/1(y = K*u) -> Sum9/2
  V/1 -> Kq/2(V), tc/4(V), PAH/1(V), Washout filter (includes forward loop below)/1(V)
  tc/1(q correc- tion) -> Sum10/2
  Sum/1 -> Sum1/1
  +/-20 deg/1 -> Sum/1
  theta-theta0/1 -> Sum/2, On/Off/2(in)
  Dthetar (PAH/GA)/1 -> Switch/3(Dthetar (PAH/RAH))

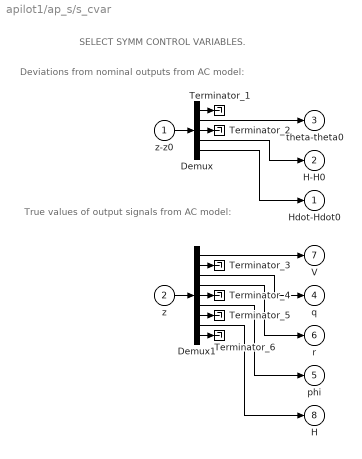
== system apilot1/ap_s/s_cvar ==
  note: SELECT SYMM CONTROL VARIABLES.
  note: True values of output
      | signals from AC model:
  note: Deviations from nominal
      | outputs from AC model:
  z-z0 : Inport  Port=1  PortWidth=-1  SampleTime=-1
  z : Inport  Port=2  PortWidth=-1  SampleTime=-1
  Demux : Demux  Outputs=[7 1 3 1 1]
  Demux1 : Demux  Outputs=[1 3 1 1 2 1 2 1 1]
  Terminator_{1..6} (6 alike) : Terminator
  Hdot-Hdot0 : Outport  Port=1  InitialOutput=0
  H-H0 : Outport  Port=2  InitialOutput=0
  theta-theta0 : Outport  Port=3  InitialOutput=0
  q : Outport  Port=4  InitialOutput=0
  phi : Outport  Port=5  InitialOutput=0
  r : Outport  Port=6  InitialOutput=0
  V : Outport  Port=7  InitialOutput=0
  H : Outport  Port=8  InitialOutput=0
  wires:
  z/1 -> Demux1/1
  Demux1/2 -> Terminator_3/1
  Demux1/5 -> Terminator_4/1
  Demux1/7 -> Terminator_5/1
  Demux1/9 -> Terminator_6/1
  Demux1/1 -> V/1
  Demux1/3 -> q/1
  Demux1/4 -> r/1
  Demux1/6 -> phi/1
  Demux1/8 -> H/1
  z-z0/1 -> Demux/1
  Demux/1 -> Terminator_1/1
  Demux/3 -> Terminator_2/1
  Demux/5 -> Hdot-Hdot0/1
  Demux/4 -> H-H0/1
  Demux/2 -> theta-theta0/1

== system apilot1/ap_s/s_mc ==
  note: SELECT SYMM MODE (on/off flags denoted by '?')
  note: SELECT SYMM REFERENCE SIGNALS
  ymode : Inport  Port=1  PortWidth=-1  SampleTime=-1
  yref : Inport  Port=2  PortWidth=-1  SampleTime=-1
  Demux : Demux  Outputs=[1 1 1 1 1 5]
  Demux1 : Demux  Outputs=[1 1 1 2]
  Terminator_1 : Terminator
  Terminator_2 : Terminator
  symm mode? : Outport  Port=1  InitialOutput=0
  symm. outer loop? : Outport  Port=2  InitialOutput=0
  Dthetar (PAH) : Outport  Port=3  InitialOutput=0
  ALS? : Outport  Port=4  InitialOutput=0
  DHdot r (ALS) : Outport  Port=5  InitialOutput=0
  ALH? : Outport  Port=6  InitialOutput=0
  DHr (ALH) : Outport  Port=7  InitialOutput=0
  GS coupled? : Outport  Port=8  InitialOutput=0
  wires:
  Demux1/3 -> DHdot r (ALS)/1
  Demux1/2 -> DHr (ALH)/1
  Demux1/1 -> Dthetar (PAH)/1
  Demux/5 -> GS coupled?/1
  Demux/4 -> ALS?/1
  Demux/3 -> ALH?/1
  Demux/1 -> symm mode?/1
  Demux/2 -> symm. outer loop?/1
  yref/1 -> Demux1/1
  Demux1/4 -> Terminator_2/1
  ymode/1 -> Demux/1
  Demux/6 -> Terminator_1/1

== system apilot1/ap_s/symm. mode ==
  crit : Inport  Port=1  PortWidth=-1  SampleTime=-1
  in : Inport  Port=2  PortWidth=-1  SampleTime=-1
  Sum : Sum  Inputs=+-
  Switch : Switch  Threshold=0
  const. : Constant  Value=0.5
  const.1 : Constant  Value=0
  out : Outport  Port=1  InitialOutput=0
  wires:
  crit/1 -> Sum/1
  const.1/1 -> Switch/3
  Sum/1 -> Switch/2
  Switch/1 -> out/1
  in/1 -> Switch/1
  const./1 -> Sum/2

== system apilot1/ap_s/t ==

== system apilot1/d+l/t ==

== system apilot1/Beaver dynamics/AC/0 ==

== system apilot1/Beaver dynamics/AC/ad ==
  x : Inport  Port=1  PortWidth=-1  SampleTime=-1
  0 : Subsystem
      settings: OpenFcn=fdchelp adgrp
      mask Display: disp('AIRDATA GROUP (level 3)\nM.O. Rauw')
  ad1 : Subsystem
      mask Type: Airdata1
      mask Description: Basic airdata variables
      mask Help: eval('fdchelp airdata1')
      mask Display: disp('Airdata1')
  ad2 : Subsystem
      mask Type: Airdata2
      mask Description: More airdata variables
      mask Help: eval('fdchelp airdata2')
      mask Display: disp('Airdata2')
  ad3 : Subsystem  mask(Airdata3){cbar=GM1(1)}
      mask prompts: cbar "Mean aerodynamic chord [m]:"
      mask help: More airdata variables
      mask Help: eval('fdchelp airdata3')
      mask Display: disp('Airdata3')
  atm : Subsystem
      mask Type: Atmosph
      mask Description: Atmosphere variables
      mask Help: eval('fdchelp atmosph')
      mask Display: disp('Atmosph')
  yatm : Outport  Port=1  InitialOutput=0
  yad1 : Outport  Port=2  InitialOutput=0
  yad2 : Outport  Port=3  InitialOutput=0
  yad3 : Outport  Port=4  InitialOutput=0
  wires:
  ad2/1(yad2) -> yad2/1
  ad3/1(yad3) -> yad3/1
  x/1 -> atm/1(x), ad1/1(x), ad3/1(x)
  atm/1(yatm) -> yatm/1, ad1/2(yatm), ad2/1(yatm), ad3/2(yatm)
  ad1/1(yad1) -> yad1/1, ad2/2(yad1), ad3/3(yad1)

== system apilot1/Beaver dynamics/AC/ae ==
  x : Inport  Port=1  PortWidth=-1  SampleTime=-1
  uaero : Inport  Port=2  PortWidth=-1  SampleTime=-1
  yad1 : Inport  Port=3  PortWidth=-1  SampleTime=-1
  0 : Subsystem
      settings: OpenFcn=fdchelp aerogrp
      mask Display: disp('AERODYNAMICS GROUP (level 3)\nM.O. Rauw')
  aero : Subsystem
      mask Type: Aeromod
      mask Description: Aerodynamic model of the DHC-2 'Beaver'.
      mask Help: eval('fdchelp aeromod')
      mask Display: disp('Aeromod\n(Beaver)')
  dl : Subsystem  mask(Dimless){cbar=GM1(1), b=GM1(2)}
      mask prompts: cbar "Mean aerodynamic chord [m]:"; b "Wing span [m]:"
      mask help: Dimensionless rotational velocities.
      mask Help: eval('fdchelp dimless')
      mask Display: disp('Dimless')
  fmdims : Subsystem  mask(FMdims){cbar=GM1(1), b=GM1(2), S=GM1(3)}
      mask prompts: cbar "Mean aerodynamic chord [m]:"; b "Wing span [m]:"; S "Wing surface [m^2]:"
      mask help:
      | Calculate forces and moments from
      | dimensionless coefficients.
      mask Help: eval('fdchelp fmdims')
      mask Display: disp('FMdims')
  ydl : Outport  Port=1  InitialOutput=0
  Caero : Outport  Port=2  InitialOutput=0
  FMaero : Outport  Port=3  InitialOutput=0
  wires:
  aero/1(Caero) -> Caero/1, fmdims/2(Force / moment coefficients)
  dl/1(ydl) -> ydl/1, aero/3(ydl)
  x/1 -> dl/1(x), aero/1(x)
  uaero/1 -> aero/2(uaero)
  yad1/1 -> fmdims/1(yad1)
  fmdims/1(Forces and moments) -> FMaero/1

== system apilot1/Beaver dynamics/AC/eng ==
  x : Inport  Port=1  PortWidth=-1  SampleTime=-1
  uprop : Inport  Port=2  PortWidth=-1  SampleTime=-1
  yatm : Inport  Port=3  PortWidth=-1  SampleTime=-1
  yad1 : Inport  Port=4  PortWidth=-1  SampleTime=-1
  0 : Subsystem
      settings: OpenFcn=fdchelp enggrp
      mask Display: disp('ENGINE GROUP (level 3)\nM.O. Rauw')
  eng : Subsystem
      mask Type: Engmod
      mask Description: Engine model for the DHC-2 'Beaver'
      mask Help: eval('fdchelp engmod')
      mask Display: disp('Engmod\n(Beaver)')
  fmdims : Subsystem  mask(FMdims){cbar=GM1(1), b=GM1(2), S=GM1(3)}
      mask prompts: cbar "Mean aerodynamic chord [m]:"; b "Wing span [m]:"; S "Wing surface [m^2]:"
      mask help:
      | Calculate forces and moments from
      | dimensionless coefficients.
      mask Help: eval('fdchelp fmdims')
      mask Display: disp('FMdims')
  pow : Subsystem
      mask Type: Power
      mask Description:
      | Engine power and dimensionless
      | pressure increase across propeller
      | (model for DHC-2 'Beaver')
      mask Help: eval('fdchelp power')
      mask Display: disp('Power\n(Beaver)')
  ypow : Outport  Port=1  InitialOutput=0
  Cprop : Outport  Port=2  InitialOutput=0
  FMprop : Outport  Port=3  InitialOutput=0
  wires:
  pow/1(ypow) -> ypow/1, eng/2(ypow)
  uprop/1 -> pow/2(uprop)
  fmdims/1(Forces and moments) -> FMprop/1
  eng/1(Cprop) -> Cprop/1, fmdims/2(Force / moment coefficients)
  yad1/1 -> fmdims/1(yad1)
  x/1 -> pow/1(x), eng/1(x)
  yatm/1 -> pow/3(yatm)

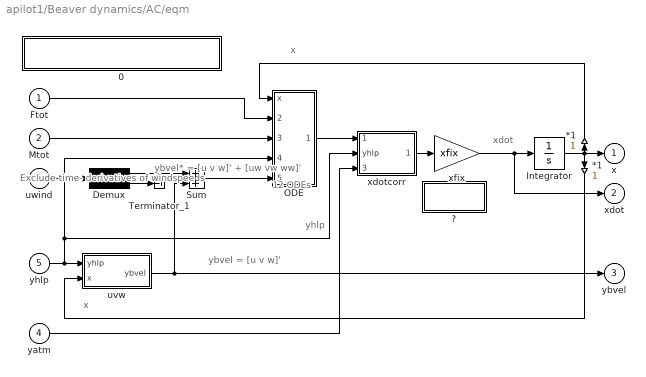
== system apilot1/Beaver dynamics/AC/eqm ==
  note: Exclude time-
      | derivatives
      | of windspeeds
  note: ybvel* =
      | [u v w]' +
      | [uw vw ww]'
  note: xdot
  note: x
  note: x
  note: yhlp
  note: ybvel = [u v w]'
  note: 12 ODEs
  Ftot : Inport  Port=1  PortWidth=-1  SampleTime=-1
  Mtot : Inport  Port=2  PortWidth=-1  SampleTime=-1
  uwind : Inport  Port=3  PortWidth=-1  SampleTime=-1
  yatm : Inport  Port=4  PortWidth=-1  SampleTime=-1
  yhlp : Inport  Port=5  PortWidth=-1  SampleTime=-1
  " *1" : Gain  Orientation=up  Gain=1
  *1 : Gain  Orientation=down  Gain=1
  0 : Subsystem
      settings: OpenFcn=fdchelp eqmotion
      mask Display: disp('EQUATIONS OF MOTION (level 3)\nM.O. Rauw')
  "?" : Subsystem
      settings: OpenFcn=fdchelp xfix
      mask Display: disp('More info\nfor xfix')
  Demux : Demux  Outputs=[3 3]
  Integrator : Integrator  ExternalReset=none  InitialConditionSource=internal  InitialCondition=xinco  LimitOutput=off  UpperSaturationLimit=inf  LowerSaturationLimit=-inf  ShowSaturationPort=off  ShowStatePort=off  AbsoluteTolerance=auto
  ODE : Subsystem
  Sum : Sum  Inputs=++
  Terminator_1 : Terminator
  uvw : Subsystem
      mask Type: uvw
      mask Description:
      | Calculation of body-axes velocities
      | u, v, and w
      mask Help: eval('fdchelp uvw')
      mask Display: disp('Body-axes\nvelocities')
  xdotcorr : Subsystem  mask(xdotcorr){b=GM1(2), S=GM1(3), m=GM1(10), CYbdot=AM(2,19)}
      mask prompts: b "Wing span [m]:"; S "Wing surface [m^2]:"; m "Mass of the aircraft [kg]:"; CYbdot "Stability-derivative CYbdot:"
      mask help:
      | Correction block to write state
      | equations for DHC-2 Beaver aircraft
      | explicitly.
      mask Help: eval('fdchelp xdotcorr')
      mask Display: disp('xdotcorr\n(Beaver)')
  xfix : Gain  Gain=xfix
  x : Outport  Port=1  InitialOutput=0
  xdot : Outport  Port=2  InitialOutput=0
  ybvel : Outport  Port=3  InitialOutput=0
  wires:
  Demux/2 -> Terminator_1/1
  yhlp/1 -> uvw/1(yhlp), ODE/4(yhlp), xdotcorr/2(yhlp)
  ODE/1(xdot) -> xdotcorr/1(xdot uncorrected)
  Sum/1 -> ODE/5(ybvel*)
  uvw/1(ybvel) -> ybvel/1, Sum/2
  uwind/1 -> Demux/1
  Demux/1 -> Sum/1
  xdotcorr/1(xdot corrected) -> xfix/1
  yatm/1 -> xdotcorr/3(yatm)
  Ftot/1 -> ODE/2(Ftot)
  Mtot/1 -> ODE/3(Mtot)
  *1/1 -> uvw/2(x)
  Integrator/1 -> x/1, " *1"/1, *1/1
  xfix/1 -> Integrator/1, xdot/1
  " *1"/1 -> ODE/1(x)

== system apilot1/Beaver dynamics/AC/fms ==
  note: `
  FMaero : Inport  Port=1  PortWidth=-1  SampleTime=-1
  FMprop : Inport  Port=2  PortWidth=-1  SampleTime=-1
  Fgrav : Inport  Port=3  PortWidth=-1  SampleTime=-1
  Fwind : Inport  Port=4  PortWidth=-1  SampleTime=-1
  0 : Subsystem
      settings: OpenFcn=fdchelp fmsort
      mask Display: disp('FMSORT\nM.O. Rauw, October 1997')
  Demux : Demux  Outputs=[3 3]
  Demux1 : Demux  Outputs=[3 3]
  Sum1 : Sum  Inputs=++
  Sum3 : Sum  Inputs=++++
  Ftot : Outport  Port=1  InitialOutput=0
  Mtot : Outport  Port=2  InitialOutput=0
  wires:
  FMaero/1 -> Demux/1
  FMprop/1 -> Demux1/1
  Demux1/2 -> Sum1/2
  Demux/2 -> Sum1/1
  Fgrav/1 -> Sum3/3
  Demux1/1 -> Sum3/2
  Sum3/1 -> Ftot/1
  Sum1/1 -> Mtot/1
  Demux/1 -> Sum3/1
  Fwind/1 -> Sum3/4

== system apilot1/Beaver dynamics/AC/fw ==
  x : Inport  Port=1  PortWidth=-1  SampleTime=-1
  uwind : Inport  Port=2  PortWidth=-1  SampleTime=-1
  -Xw/m : Fcn  Expr=u[16] + u[5]*u[15] - u[6]*u[14]
  -Yw/m : Fcn  Expr=u[17] - u[4]*u[15] + u[6]*u[13]
  -Zw/m : Fcn  Expr=u[18] + u[4]*u[14] - u[5]*u[13]
  0 : Subsystem
      settings: OpenFcn=fdchelp fwind
      mask Display: disp('FWIND\nM.O. Rauw, Dec. 1996')
  Mux : Mux  Inputs=3
  Mux1 : Mux  Inputs=[12 6]
  gain : Gain  Gain=-m
  Fwind : Outport  Port=1  InitialOutput=0
  wires:
  uwind/1 -> Mux1/2
  x/1 -> Mux1/1
  gain/1 -> Fwind/1
  Mux/1 -> gain/1
  Mux1/1 -> -Yw/m/1, -Zw/m/1, -Xw/m/1
  -Yw/m/1 -> Mux/2
  -Xw/m/1 -> Mux/1
  -Zw/m/1 -> Mux/3

== system apilot1/Beaver dynamics/AC/gr ==
  x : Inport  Port=1  PortWidth=-1  SampleTime=-1
  yatm : Inport  Port=2  PortWidth=-1  SampleTime=-1
  0 : Subsystem
      settings: OpenFcn=fdchelp gravity
      mask Display: disp('GRAVITY\nM.O. Rauw, October 1997')
  Mux : Mux  Inputs=3
  Mux1 : Mux  Inputs=[12 5]
  Xgr : Fcn  Expr=-m*u[17]*sin(u[8])
  Ygr : Fcn  Expr=m*u[17]*cos(u[8])*sin(u[9])
  Zgr : Fcn  Expr=m*u[17]*cos(u[8])*cos(u[9])
  Fgrav : Outport  Port=1  InitialOutput=0
  wires:
  Xgr/1 -> Mux/1
  Ygr/1 -> Mux/2
  Mux/1 -> Fgrav/1
  Mux1/1 -> Ygr/1, Xgr/1, Zgr/1
  Zgr/1 -> Mux/3
  x/1 -> Mux1/1
  yatm/1 -> Mux1/2

== system apilot1/Beaver dynamics/AC/hlp ==
  note: '
  x : Inport  Port=1  PortWidth=-1  SampleTime=-1
  0 : Subsystem
      settings: OpenFcn=fdchelp hlpfcn
      mask Display: disp('HELP FUNCTIONS\n(often used sines and cosines)\nM.O. Rauw, October 1997')
  Mux : Mux  Inputs=11
  cos alpha : Fcn  Expr=cos(u[2])
  cos beta : Fcn  Expr=cos(u[3])
  cos phi : Fcn  Expr=cos(u[9])
  cos psi : Fcn  Expr=cos(u[7])
  cos theta : Fcn  Expr=cos(u[8])
  sin alpha : Fcn  Expr=sin(u[2])
  sin beta : Fcn  Expr=sin(u[3])
  sin phi : Fcn  Expr=sin(u[9])
  sin psi : Fcn  Expr=sin(u[7])
  sin theta : Fcn  Expr=sin(u[8])
  tan beta : Fcn  Expr=tan(u[3])
  yhlp : Outport  Port=1  InitialOutput=0
  wires:
  x/1 -> sin psi/1, sin beta/1, cos beta/1, sin alpha/1, cos alpha/1, tan beta/1, sin theta/1, cos theta/1, sin phi/1, cos phi/1, cos psi/1
  cos alpha/1 -> Mux/1
  sin alpha/1 -> Mux/2
  cos beta/1 -> Mux/3
  sin beta/1 -> Mux/4
  tan beta/1 -> Mux/5
  sin psi/1 -> Mux/6
  cos psi/1 -> Mux/7
  sin theta/1 -> Mux/8
  cos theta/1 -> Mux/9
  sin phi/1 -> Mux/10
  Mux/1 -> yhlp/1
  cos phi/1 -> Mux/11

== system apilot1/Beaver dynamics/AC/out ==
  note: Flightpath
      | variables
  note: du/dt, dv/dt, dw/dt
      | (output equations!)
  note: Body-axes accelerations
      | and specific forces
  x : Inport  Port=1  PortWidth=-1  SampleTime=-1
  xdot : Inport  Port=2  PortWidth=-1  SampleTime=-1
  yhlp : Inport  Port=3  PortWidth=-1  SampleTime=-1
  Ftot : Inport  Port=4  PortWidth=-1  SampleTime=-1
  Fgrav : Inport  Port=5  PortWidth=-1  SampleTime=-1
  0 : Subsystem
      settings: OpenFcn=fdchelp moreouts
      mask Display: disp('Additional outputs (level 3)\nM.O. Rauw')
  accel : Subsystem  mask(accel){m=GM1(10)}
      mask prompts: m "Mass of the aircraft [kg]:"
      mask help:
      | Body axes accelerations and
      | specific forces.
      mask Help: eval('fdchelp accel')
      mask Display: disp('Accel')
  fp : Subsystem  mask(Flpath){alpha0=xinco(2)}
      mask prompts: alpha0 "Initial value of angle of attack, alpha0:"
      mask help: Flightpath related parameters.
      mask Help: eval('fdchelp flpath')
      mask Display: disp('flpath')
  uvwdot : Subsystem
      mask Type: uvwdot
      mask Description: Calculation of du/dt, dv/dt, and dw/dt.
      mask Help: eval('fdchelp uvwdot')
      mask Display: disp('uvwdot')
  yfp : Outport  Port=1  InitialOutput=0
  yuvw : Outport  Port=2  InitialOutput=0
  yacc : Outport  Port=3  InitialOutput=0
  wires:
  fp/1(yfp) -> yfp/1
  uvwdot/1(yuvw =  [udot; vdot; wdot]) -> yuvw/1
  yhlp/1 -> uvwdot/3(yhlp)
  Ftot/1 -> accel/1(Ftot)
  accel/1(yacc) -> yacc/1
  xdot/1 -> fp/2(xdot), uvwdot/2(xdot)
  x/1 -> fp/1(x), uvwdot/1(x)
  Fgrav/1 -> accel/2(Fgrav)

== system apilot1/ap_as/HH/Kpsi ==
  V : Inport  Port=1  PortWidth=-1  SampleTime=-1
  input u : Inport  Port=2  PortWidth=-1  SampleTime=-1
  Kpsi(V) : Fcn  Expr=0.05*u[1] - 1.1
  Product : Product  Inputs=2
  y = K*u : Outport  Port=1  InitialOutput=0
  wires:
  Kpsi(V)/1 -> Product/1
  input u/1 -> Product/2
  Product/1 -> y = K*u/1
  V/1 -> Kpsi(V)/1

== system apilot1/ap_as/HH/On/Off ==
  crit : Inport  Port=1  PortWidth=-1  SampleTime=-1
  in : Inport  Port=2  PortWidth=-1  SampleTime=-1
  Sum : Sum  Inputs=+-
  Switch : Switch  Threshold=0
  const. : Constant  Value=0.5
  const.1 : Constant  Value=0
  out : Outport  Port=1  InitialOutput=0
  wires:
  const./1 -> Sum/2
  in/1 -> Switch/1
  Switch/1 -> out/1
  Sum/1 -> Switch/2
  const.1/1 -> Switch/3
  crit/1 -> Sum/1

== system apilot1/ap_as/RAH/Kr*(g/V) ==
  input u : Inport  Port=1  PortWidth=-1  SampleTime=-1
  V : Inport  Port=2  PortWidth=-1  SampleTime=-1
  Kr*(g/V) : Fcn  Expr=-4*(9.80665/u[1])
  Product : Product  Inputs=2
  y = K*u : Outport  Port=1  InitialOutput=0
  wires:
  V/1 -> Kr*(g/V)/1
  Product/1 -> y = K*u/1
  input u/1 -> Product/2
  Kr*(g/V)/1 -> Product/1

== system apilot1/ap_as/RAH/RAH ==
  note: PI controller for RAH
  V : Inport  Port=1  PortWidth=-1  SampleTime=-1
  input u : Inport  Port=2  PortWidth=-1  SampleTime=-1
  +/-1V : Integrator  ExternalReset=none  InitialConditionSource=internal  InitialCondition=0  LimitOutput=on  UpperSaturationLimit=1*pi/180  LowerSaturationLimit=-1*pi/180  ShowSaturationPort=off  ShowStatePort=off  AbsoluteTolerance=auto
  +/-3.75V : Saturate  UpperLimit=3.75*pi/180  LowerLimit=-3.75*pi/180
  Ki : Gain  Gain=0.25
  Kphi : Subsystem
      mask Display: plot(0,0,100,100,[0,100,0],[0,50,100]);disp('K(u1)      ')
  Sum : Sum  Inputs=++
  output y : Outport  Port=1  InitialOutput=0
  wires:
  input u/1 -> Kphi/2(input u)
  Kphi/1(y = K*u) -> +/-3.75V/1
  V/1 -> Kphi/1(V)
  +/-3.75V/1 -> Ki/1, Sum/1
  +/-1V/1 -> Sum/2
  Ki/1 -> +/-1V/1
  Sum/1 -> output y/1

== system apilot1/ap_as/RAH/Switch ==
  Dphir (out. loop) : Inport  Port=1  PortWidth=-1  SampleTime=-1
  Asymm.  out. loop? : Inport  Port=2  PortWidth=-1  SampleTime=-1
  Dphir (RAH) : Inport  Port=3  PortWidth=-1  SampleTime=-1
  Sum2 : Sum  Inputs=-+
  Switch : Switch  Threshold=0
  const : Constant  Value=0.5
  Dphir : Outport  Port=1  InitialOutput=0
  wires:
  Dphir (out. loop)/1 -> Switch/1
  Dphir (RAH)/1 -> Switch/3
  Sum2/1 -> Switch/2
  const/1 -> Sum2/1
  Switch/1 -> Dphir/1
  Asymm.  out. loop?/1 -> Sum2/2

== system apilot1/ap_as/RAH/drr-Kr ==
  input u : Inport  Port=1  PortWidth=-1  SampleTime=-1
  V : Inport  Port=2  PortWidth=-1  SampleTime=-1
  Product : Product  Inputs=2
  drr-Kr : Fcn  Expr=(-7.5*10^(-5)*u[1]^2 + 0.0095*u[1] - 0.4606) + 4
  y = K*u : Outport  Port=1  InitialOutput=0
  wires:
  drr-Kr/1 -> Product/1
  Product/1 -> y = K*u/1
  V/1 -> drr-Kr/1
  input u/1 -> Product/2

== system apilot1/ap_s/ALH/KH ==
  V : Inport  Port=1  PortWidth=-1  SampleTime=-1
  input u : Inport  Port=2  PortWidth=-1  SampleTime=-1
  KH(V) : Fcn  Expr=(-1.0*10^(-4)*u[1]^2 + 0.015*u[1] - 0.5975)*(pi/180)
  Product : Product  Inputs=2
  y = K*u : Outport  Port=1  InitialOutput=0
  wires:
  V/1 -> KH(V)/1
  Product/1 -> y = K*u/1
  input u/1 -> Product/2
  KH(V)/1 -> Product/1

== system apilot1/ap_s/ALH/On/Off ==
  crit : Inport  Port=1  PortWidth=-1  SampleTime=-1
  in : Inport  Port=2  PortWidth=-1  SampleTime=-1
  Sum : Sum  Inputs=+-
  Switch : Switch  Threshold=0
  const. : Constant  Value=0.5
  const.1 : Constant  Value=0
  out : Outport  Port=1  InitialOutput=0
  wires:
  const./1 -> Sum/2
  in/1 -> Switch/1
  Switch/1 -> out/1
  Sum/1 -> Switch/2
  const.1/1 -> Switch/3
  crit/1 -> Sum/1

== system apilot1/ap_s/ALS/KHdot ==
  V : Inport  Port=1  PortWidth=-1  SampleTime=-1
  input u : Inport  Port=2  PortWidth=-1  SampleTime=-1
  KHdot(V) : Fcn  Expr=(-3.875*10^(-4)*u[1]^2 + 0.04025*u[1] - 1.1041)*(pi/180)
  Product : Product  Inputs=2
  y = K*u : Outport  Port=1  InitialOutput=0
  wires:
  KHdot(V)/1 -> Product/1
  input u/1 -> Product/2
  Product/1 -> y = K*u/1
  V/1 -> KHdot(V)/1

== system apilot1/ap_s/ALS/On/Off ==
  crit : Inport  Port=1  PortWidth=-1  SampleTime=-1
  in : Inport  Port=2  PortWidth=-1  SampleTime=-1
  Sum : Sum  Inputs=+-
  Switch : Switch  Threshold=0
  const. : Constant  Value=0.5
  const.1 : Constant  Value=0
  out : Outport  Port=1  InitialOutput=0
  wires:
  crit/1 -> Sum/1
  const.1/1 -> Switch/3
  Sum/1 -> Switch/2
  Switch/1 -> out/1
  in/1 -> Switch/1
  const./1 -> Sum/2

== system apilot1/ap_s/PAH/Kq ==
  input u : Inport  Port=1  PortWidth=-1  SampleTime=-1
  V : Inport  Port=2  PortWidth=-1  SampleTime=-1
  Kq(V) : Fcn  Expr=-4.75*10^(-4)*u[1]^2 +0.0540*u[1] - 1.5931
  Product : Product  Inputs=2
  y = K*u : Outport  Port=1  InitialOutput=0
  wires:
  V/1 -> Kq(V)/1
  Product/1 -> y = K*u/1
  input u/1 -> Product/2
  Kq(V)/1 -> Product/1

== system apilot1/ap_s/PAH/On/Off ==
  crit. : Inport  Port=1  PortWidth=-1  SampleTime=-1
  in : Inport  Port=2  PortWidth=-1  SampleTime=-1
  Sum : Sum  Inputs=+-
  Switch : Switch  Threshold=0
  const. : Constant  Value=0.5
  const.1 : Constant  Value=0
  out : Outport  Port=1  InitialOutput=0
  wires:
  crit./1 -> Sum/1
  const.1/1 -> Switch/3
  Sum/1 -> Switch/2
  Switch/1 -> out/1
  in/1 -> Switch/1
  const./1 -> Sum/2
